simulink model "FSK"  (R2020b)
settings: Solver=VariableStepAuto  StartTime=0.0  StopTime=10.0  RelTol=1e-3
settings Model: Creator=LENOVO  LastModifiedBy=LENOVO

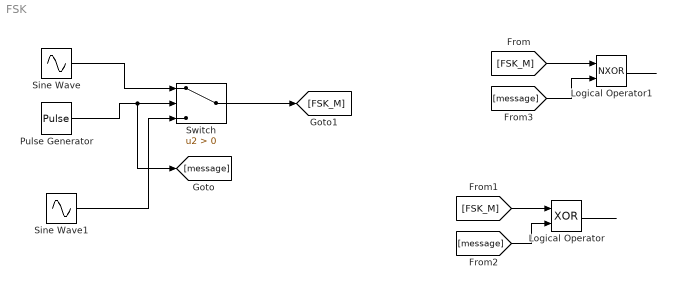
== system FSK ==
  Logical Operator : Logic  Operator=XOR  AllPortsSameDT=off  OutDataTypeStr=boolean
  Logical Operator1 : Logic  Operator=NXOR  AllPortsSameDT=off  OutDataTypeStr=boolean
  Pulse Generator : DiscretePulseGenerator  PulseType=Time based  Period=10  PulseWidth=5
  Sine Wave : Sin  Amplitude=5  Frequency=2*pi*15000  Phase=90  SampleTime=0.02
  Sine Wave1 : Sin  Amplitude=5  Frequency=2*pi*25000  SampleTime=0.02
  Switch : Switch  Criteria=u2 > Threshold
  wires:
  Sine Wave/1 -> Switch/1
  Pulse Generator/1 -> [message], Switch/2
  Sine Wave1/1 -> Switch/3
  Switch/1 -> [FSK_M]
  [FSK_M] -> Logical Operator/1
  [FSK_M] -> Logical Operator1/1
  [message] -> Logical Operator1/2
  [message] -> Logical Operator/2
  Logical Operator/1 -> ?
  Logical Operator1/1 -> ?
